simulink model "DTDSM_1b_2or_512osr"  (R2019b)
settings: Solver=VariableStepAuto  StartTime=0.0  StopTime=ts*(Mpoints+10)  RelTol=1e-3
InitFcn:
  | %fs=256*2e4;
  | %osr=512;
  | ts=1/fs;
  | 
  | Ncycle=37;
  | Mpoints=2^16;
  | fin=fs*Ncycle/Mpoints;
  | 
  | 
  | ref=2;
values from neighbouring files (symbols this model uses):
  fs = osr*2e4    (= 10240000)    [CTSDM.m]
  osr = 512    [CTSDM.m]    (also in ENOB.m = logspace(log10(64), log10(2^15), 1000); SNR.m = logspace(log10(64), log10(2^15), 1000))
undefined symbols (not defined in the file or in its folder): a1, argo, b1, c1, g1
libraries: SDtoolbox x4
settings Model: Creator=lenovo  LastModifiedBy=lenovo

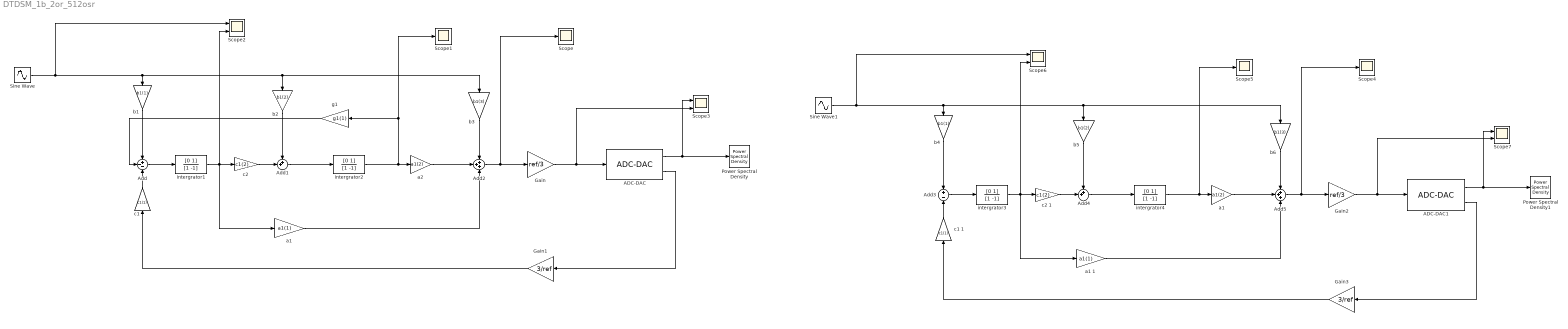
== system DTDSM_1b_2or_512osr ==
  ADC-DAC : SDtoolbox/ADC-DAC  k=1  MM=off  match=0  CST=0  VVG=off  argo=argo(:,3)  LF=on  NF=retA.log
      settings: SourceProductName=SDtoolbox
  ADC-DAC1 : SDtoolbox/ADC-DAC  k=1  MM=off  match=0  CST=0  VVG=off  argo=argo(:,3)  LF=on  NF=retA.log
      settings: SourceProductName=SDtoolbox
  Add : Sum  Inputs=+--
  Add1 : Sum  Inputs=++|
  Add2 : Sum  Inputs=+++
  Add3 : Sum  Inputs=+|-
  Add4 : Sum  Inputs=++|
  Add5 : Sum  Inputs=+++
  Gain : Gain  Gain=ref/3
  Gain1 : Gain  Gain=3/ref
  Gain2 : Gain  Gain=ref/3
  Gain3 : Gain  Gain=3/ref
  Power Spectral Density : SDtoolbox/Power Spectral Density  SN=1  Fs=fs  fBL=1  fBH=fs/(2*osr)  Fin=fin  N=Mpoints  Ntransient=10  VW=off  savename=savemat  Scale_type=logarithmic
      settings: SourceProductName=SDtoolbox
  Power Spectral Density1 : SDtoolbox/Power Spectral Density  SN=2  Fs=fs  fBL=1  fBH=fs/(2*osr)  Fin=fin  N=Mpoints  Ntransient=10  VW=off  savename=savemat  Scale_type=logarithmic
      settings: SourceProductName=SDtoolbox
  Scope{,1,4..5} (4 alike) : Scope
  Scope{2..3,6..7} (4 alike) : Scope  NumInputPorts=2
  Sine Wave : Sin  Amplitude=1.1  Frequency=fin*2*pi  SampleTime=ts
  Sine Wave1 : Sin  Amplitude=1.1  Frequency=fin*2*pi  SampleTime=ts
  a1 : Gain  Gain=a1(2)
  "a1 " : Gain  Gain=a1(1)
  a1 1 : Gain  Gain=a1(1)
  a2 : Gain  Gain=a1(2)
  b1 : Gain  Gain=b1(1)
  b2 : Gain  Gain=b1(2)
  b3 : Gain  Gain=b1(3)
  b4 : Gain  Gain=b1(1)
  b5 : Gain  Gain=b1(2)
  b6 : Gain  Gain=b1(3)
  "c1 " : Gain  Gain=c1(1)
  c1 1 : Gain  Gain=c1(1)
  "c2 " : Gain  Gain=c1(2)
  c2 1 : Gain  Gain=c1(2)
  g1 : Gain  Gain=g1(1)
  intergrator{1..4} (4 alike) : DiscreteFilter  Numerator=[0 1]  Denominator=[1 -1]
  wires:
  Sine Wave/1 -> Scope2/1, b3/1, b2/1, b1/1
  b1/1 -> Add/1
  Add/1 -> intergrator1/1
  "c1 "/1 -> Add/3
  b2/1 -> Add1/1
  "c2 "/1 -> Add1/2
  intergrator1/1 -> Scope2/2, "a1 "/1, "c2 "/1
  Add1/1 -> intergrator2/1
  a2/1 -> Add2/2
  intergrator2/1 -> Scope1/1, g1/1, a2/1
  "a1 "/1 -> Add2/3
  b3/1 -> Add2/1
  g1/1 -> Add/2
  Gain1/1 -> "c1 "/1
  Gain/1 -> Scope3/2, ADC-DAC/1
  Add2/1 -> Scope/1, Gain/1
  ADC-DAC/2 -> Gain1/1
  ADC-DAC/1 -> Scope3/1, Power Spectral Density/1
  Gain3/1 -> c1 1/1
  b5/1 -> Add4/1
  ADC-DAC1/1 -> Scope7/1, Power Spectral Density1/1
  a1 1/1 -> Add5/3
  intergrator3/1 -> Scope6/2, a1 1/1, c2 1/1
  Add3/1 -> intergrator3/1
  Add5/1 -> Scope4/1, Gain2/1
  Gain2/1 -> Scope7/2, ADC-DAC1/1
  a1/1 -> Add5/2
  c1 1/1 -> Add3/2
  Add4/1 -> intergrator4/1
  c2 1/1 -> Add4/2
  intergrator4/1 -> Scope5/1, a1/1
  ADC-DAC1/2 -> Gain3/1
  b6/1 -> Add5/1
  b4/1 -> Add3/1
  Sine Wave1/1 -> Scope6/1, b6/1, b5/1, b4/1
